simulink model "schemat"  (R2022b)
settings: Solver=VariableStepAuto  StartTime=0.0  StopTime=10.0  RelTol=1e-3
values from neighbouring files (symbols this model uses):
  A = [0,       1,             0, 0 ... (first row only)    [main.m]
  B = [0, 1/M, 0, 1/(M*L)]'    [main.m]
  C = eye(4)    [main.m]
  D = [0, 0, 0,0]'    [main.m]
  K = lqr(system, Q, R)    [main.m]
  Y = [y, 0, 0, 0]'    [main.m]
libraries: eeLuenbergerObserver x1
settings Model: Creator=asialalala  LastModifiedBy=asialalala
settings DataIOCC: ReturnWorkspaceOutputs=off

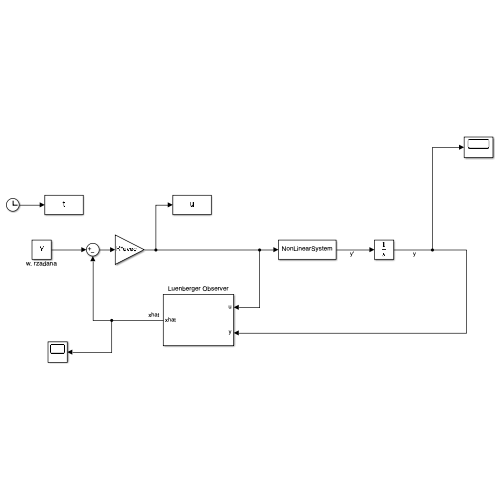
[thumbnail: Simulink's stored preview of the top-level diagram]
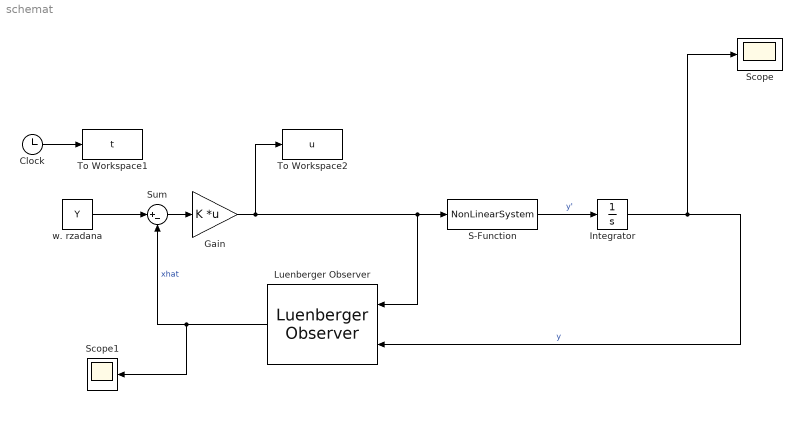
== system schemat ==
  Clock : Clock
  Gain : Gain  Gain=K  Multiplication=Matrix(K*u) (u vector)
  Integrator : Integrator
  Luenberger Observer : eeLuenbergerObserver/Luenberger Observer  StateSpaceType=Continuous-time  Ad=A  Bd=b  Cd=C  Dd=D  A=A  B=B  C=C  D=D  ObserverDesign=Observer gain  Ld=2  DesiredEigenvalues=lambda  x0=state0  Tsd=0.1  Ts=0.001
  S-Function : S-Function  FunctionName=NonLinearSystem  Parameters=state0, params  SFunctionDeploymentMode=off  EnableBusSupport=off
  Scope : Scope
  Scope1 : Scope
  Sum : Sum  Inputs=|+-
  To Workspace1 : ToWorkspace  VariableName=t  SampleTime=-1
  To Workspace2 : ToWorkspace  VariableName=u  SampleTime=-1
  w. rzadana : Constant  Value=Y
  wires:
  Sum/1 -> Gain/1
  S-Function/1 -> Integrator/1  "y'"
  w. rzadana/1 -> Sum/1
  Gain/1 -> To Workspace2/1, Luenberger Observer/1, S-Function/1
  Clock/1 -> To Workspace1/1
  Luenberger Observer/1 -> Scope1/1, Sum/2  "xhat"
  Integrator/1 -> Scope/1, Luenberger Observer/2  "y"
